simulink model "noxiebo"  (R2018b)
settings: Solver=FixedStepDiscrete  StartTime=0.0  StopTime=Inf  FixedStep=Auto  RelTol=1e-3  EnableMultiTasking=on
model workspace (MAT data in the model file):
  encoderResolution = 4096
  indexOffset = 0
  polePairs = 16
undefined symbols (not defined in the file or in its folder): Down, Up
libraries: idelinklib_common x37, c2833xlib x7, c280xlib x6, simulink x3, simulink_extras x2, c2000lib x1
(part 1 of 3)
settings Model: ExtModeTrigDuration=8  Creator=ChenYu  LastModifiedBy=ThinkPad
settings DataIOCC: LimitDataPoints=on  SaveFormat=Array  SignalLoggingSaveFormat=ModelDataLogs  SaveOutput=off  SaveTime=off
settings OptimizationCC: DefaultUnderspecifiedDataType=single  EnhancedBackFolding=on  PassReuseOutputArgsAs=Individual arguments  ExpressionDepthLimit=2147483647  MaxStackSize=512  OptimizeBlockOrder=speed  DifferentSizesBufferReuse=on  OptimizationCustomize=off
settings DebuggingCC: UnderspecifiedInitializationDetection=Classic  MergeDetectMultiDrivingBlocksExec=none  SolverPrmCheckMsg=warning  ParameterTunabilityLossMsg=error  FcnCallInpInsideContextMsg=warning  StateNameClashWarn=warning  SFUnexpectedBacktrackingDiag=warning  SFNoUnconditionalDefaultTransitionDiag=warning  SFExecutionAtInitializationDiag=none
settings HardwareCC: ProdBitPerChar=16  ProdBitPerInt=16  ProdBitPerPointer=32  ProdBitPerSizeT=32  ProdBitPerPtrDiffT=32  ProdLargestAtomicInteger=Integer  ProdLargestAtomicFloat=None  ProdWordSize=16  ProdLongLongMode=on  ProdHWDeviceType=Texas Instruments->C2000
settings ModelReferenceCC: PropagateSignalLabelsOutOfModel=off
settings SFSimCC: SimUseLocalCustomCode=off  MATLABDynamicMemAlloc=off
settings RTWCC: SystemTargetFile=ert.tlc  HardwareBoard=TI Delfino F2833x  GenCodeOnly=on  TemplateMakefile=ert_default_tmf  GenerateReport=on  RTWUseLocalCustomCode=off  Toolchain=Texas Instruments Code Composer Studio (C2000)  IncludeHyperlinkInReport=on  LaunchReport=on  GenerateTraceInfo=on  GenerateTraceReport=on  GenerateTraceReportSl=on  GenerateTraceReportSf=on  GenerateTraceReportEml=on
settings RTWCC: CustomInitializer=|
  | // Make sure the XINTF clock is enabled   cool
  | 	SysCtrlRegs.PCLKCR3.bit.XINTFENCLK = 1;
  | 
  | 	// Configure the GPIO for XINTF with a 16-bit data bus
  | 	// This function is in DSP2833x_Xintf.c
  | 	//InitXintf16Gpio();
  | 
  |     EALLOW;
  |     // All Zones---------------------------------
  |     // Timing for all zones based on XTIMCLK = SYSCLKOUT/2
  |     XintfRegs.XINTCNF2.bit.XTIMCLK = 1;
  |     // Buffer up to 3 writes
  |     XintfRegs.XINTCNF2.bit.WRBUFF = 3;
  |     // XCLKOUT is enabled
  |     XintfRegs.XINTCNF2.bit.CLKOFF = 0;
  |     // XCLKOUT = XTIMCLK/2
  |     XintfRegs.XINTCNF2.bit.CLKMODE = 1;
  | 
  |     // Zone 7------------------------------------
  |     // When using ready, ACTIVE must be 1 or greater
  |     // Lead must always be 1 or greater
  |     // Zone write timing
  |     XintfRegs.XTIMING7.bit.XWRLEAD = 3;//3*2*2*SYSCLKOUT
  |     XintfRegs.XTIMING7.bit.XWRACTIVE = 7; //(7+1)*2*2*SYSCLKOUT
  |     XintfRegs.XTIMING7.bit.XWRTRAIL = 3;
  |     // Zone read timing
  |     XintfRegs.XTIMING7.bit.XRDLEAD = 3;
  |     XintfRegs.XTIMING7.bit.XRDACTIVE = 7;
  |     XintfRegs.XTIMING7.bit.XRDTRAIL = 3;
  | 
  |     // double all Zone read/write lead/active/trail timing
  |     XintfRegs.XTIMING7.bit.X2TIMING = 1;
  | 
  |     // Zone will not sample XREADY signal
  |     XintfRegs.XTIMING7.bit.USEREADY = 0;
  |     XintfRegs.XTIMING7.bit.READYMODE = 0;
  | 
  |     // Size must be either:
  |     // 0,1 = x32 or
  |     // 1,1 = x16 other values are reserved
  |     XintfRegs.XTIMING7.bit.XSIZE = 3;
  | 
  |     EDIS;
  | 
  |    //Force a pipeline flush to ensure that the write to
  |    //the last register configured occurs before returning.
  |    asm(" RPT #7 || NOP");
settings CodeAppCC: ForceParamTrailComments=on  IgnoreCustomStorageClasses=off  OperatorAnnotations=on  SimulinkDataObjDesc=on  SFDataObjDesc=on  CustomSymbolStrType=$N$R$M  InsertBlockDesc=on  InternalIdentifier=Classic
settings ERTTargetCC: CodeReplacementLibrary=TI C28x
settings ConfigComp: CovMetricSettings=dw  CovHtmlReporting=on  CovSaveCumulativeToWorkspaceVar=on  CovSaveSingleToWorkspaceVar=on  CovExternalEMLEnable=off

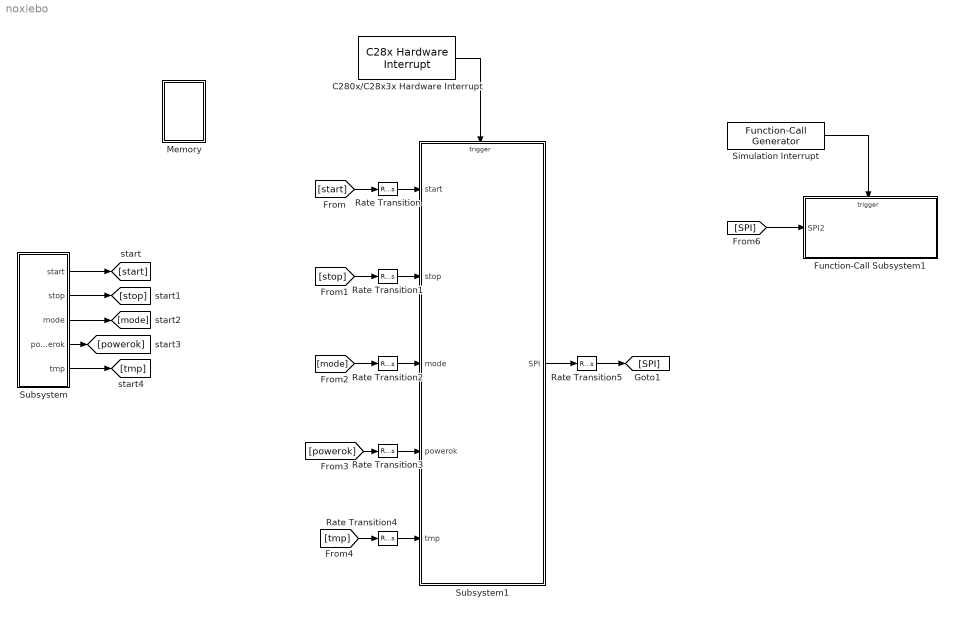
== system noxiebo ==
  C280x/C28x3x Hardware Interrupt : c2000lib/Scheduling/C28x Hardware Interrupt  irqnumbers=[3]  pienumbers=[1]  irqpriorities=[30]  irqpreempts=[0]  showinput=off  dspchiptype=C280X
      settings: SourceProductName=Embedded Coder Support Package for Texas Instruments C2000 Processors  SourceProductBaseCode=TIC2000
  Function-Call Subsystem1 : Subsystem  TreatAsAtomicUnit=on
  Memory : Subsystem
  Rate Transition{,1..5} (6 alike) : RateTransition  Integrity=off
  Simulation Interrupt : simulink/Ports & Subsystems/Function-Call Generator  sample_time=0.005  numberOfIterations=1
  Subsystem : Subsystem
  Subsystem1 : Subsystem
  wires:
  Subsystem/1(start) -> [start]
  Subsystem/2(stop) -> [stop]
  Subsystem/3(mode) -> [mode]
  Subsystem/4(powerok) -> [powerok]
  Subsystem/5(tmp) -> [tmp]
  [start] -> Rate Transition/1
  [stop] -> Rate Transition1/1
  [mode] -> Rate Transition2/1
  [powerok] -> Rate Transition3/1
  [tmp] -> Rate Transition4/1
  Rate Transition/1 -> Subsystem1/1(start)
  Rate Transition1/1 -> Subsystem1/2(stop)
  Rate Transition2/1 -> Subsystem1/3(mode)
  Rate Transition3/1 -> Subsystem1/4(powerok)
  C280x/C28x3x Hardware Interrupt/1 -> Subsystem1/Trigger
  Rate Transition4/1 -> Subsystem1/5(tmp)
  [SPI] -> Function-Call Subsystem1/1(SPI2)
  Simulation Interrupt/1 -> Function-Call Subsystem1/Trigger
  Rate Transition5/1 -> [SPI]
  Subsystem1/1(SPI) -> Rate Transition5/1

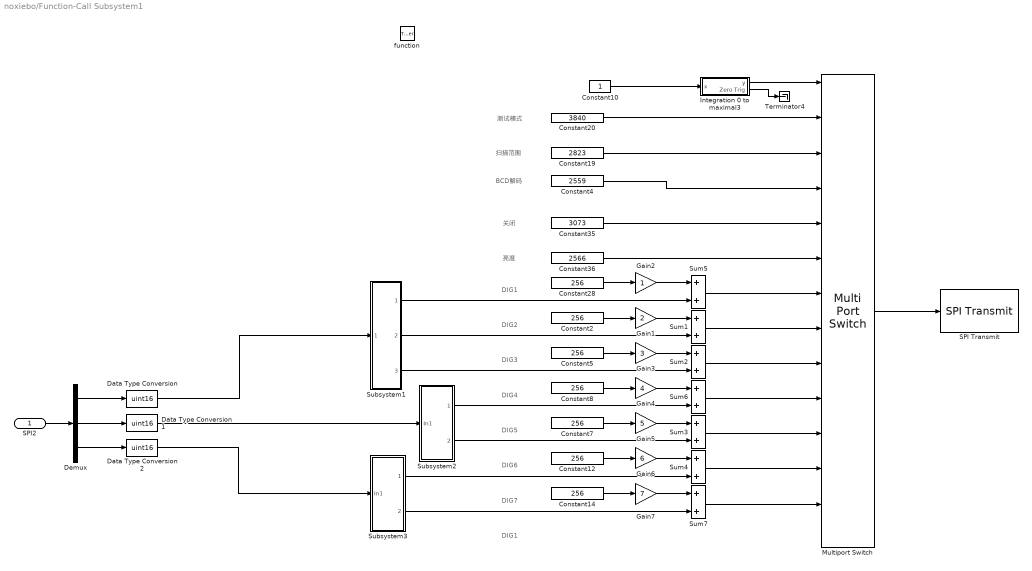
== system noxiebo/Function-Call Subsystem1 ==
  note: 扫描范围
  note: 测试模式
  note: BCD解码
  note: 关闭
  note: 亮度
  note: DIG1
  note: DIG2
  note: DIG3
  note: DIG4
  note: DIG5
  note: DIG6
  note: DIG7
  note: DIG1
  SPI2 : Inport
  function : TriggerPort  TriggerType=function-call  VariantControl=(inherit)
  Constant10 : Constant  OutDataTypeStr=uint16
  Constant{2,5,7..8,12,14,28} (7 alike) : Constant  Value=256  OutDataTypeStr=uint16
  Constant19 : Constant  Value=2823  OutDataTypeStr=uint16
  Constant20 : Constant  Value=3840  OutDataTypeStr=uint16
  Constant35 : Constant  Value=3073  OutDataTypeStr=uint16
  Constant36 : Constant  Value=2566  OutDataTypeStr=uint16
  Constant4 : Constant  Value=2559  OutDataTypeStr=uint16
  Data Type Conversion : DataTypeConversion  OutDataTypeStr=uint16
  Data Type Conversion1 : DataTypeConversion  OutDataTypeStr=uint16
  Data Type Conversion2 : DataTypeConversion  OutDataTypeStr=uint16
  Demux : Demux  Outputs=3
  Gain1 : Gain  Gain=2
  Gain2 : Gain
  Gain3 : Gain  Gain=3
  Gain4 : Gain  Gain=4
  Gain5 : Gain  Gain=5
  Gain6 : Gain  Gain=6
  Gain7 : Gain  Gain=7
  Integration 0 to maximal3 : Subsystem  mask{a=12}
      mask prompts: a "the maximal y"
  Multiport Switch : MultiPortSwitch  Inputs=12  DataPortForDefault=Additional data port  OutDataTypeStr=uint16
  SPI Transmit : c280xlib/SPI Transmit  SPISelect=SPI_A  ClockPolarity=Rising_edge  ClockPhase=No_delay  SPIModule=uint32(0)  Mode=Master  BusSpeed=uint32(1000000)  FirstBitToTransfer=Most significant bit (MSB)  ClockMode=0  BlockFunction=Write  EnableRegisterAddress=on  RegisterAddress=0  OutputDataType=int8  OutputDataLength=1  BlockingMode=off  DataBits=8  UseCustomSSPin=Provided by the SPI peripheral  ActiveLowSSPin=Active low  Pin=0
      settings: SourceProductName=Embedded Coder Support Package for Texas Instruments C2000 Processors  SourceProductBaseCode=TIC2000
  Subsystem1 : Subsystem
  Subsystem2 : Subsystem
  Subsystem3 : Subsystem
  Sum{1..7} (7 alike) : Sum
  Terminator4 : Terminator
  wires:
  Constant10/1 -> Integration 0 to maximal3/1(x)
  Constant19/1 -> Multiport Switch/3
  Constant20/1 -> Multiport Switch/2
  Integration 0 to maximal3/1(y) -> Multiport Switch/1
  Constant35/1 -> Multiport Switch/5
  Constant36/1 -> Multiport Switch/6
  Multiport Switch/1 -> SPI Transmit/1
  Constant28/1 -> Gain2/1
  Sum5/1 -> Multiport Switch/7
  Constant2/1 -> Gain1/1
  Sum1/1 -> Multiport Switch/8
  Constant5/1 -> Gain3/1
  Sum2/1 -> Multiport Switch/9
  Sum6/1 -> Multiport Switch/10
  Subsystem2/1(Out2) -> Sum6/2
  Constant7/1 -> Gain5/1
  Sum3/1 -> Multiport Switch/11
  Subsystem2/2(Out3) -> Sum3/2
  Constant12/1 -> Gain6/1
  Sum4/1 -> Multiport Switch/12
  Subsystem3/1(Out2) -> Sum4/2
  Constant14/1 -> Gain7/1
  Sum7/1 -> Multiport Switch/13
  Gain2/1 -> Sum5/1
  Constant8/1 -> Gain4/1
  Gain1/1 -> Sum1/1
  Gain3/1 -> Sum2/1
  Gain4/1 -> Sum6/1
  Gain5/1 -> Sum3/1
  Gain6/1 -> Sum4/1
  Subsystem3/2(Out3) -> Sum7/2
  Gain7/1 -> Sum7/1
  Constant4/1 -> Multiport Switch/4
  Subsystem1/1(Out1) -> Sum5/2
  Subsystem1/2(Out2) -> Sum1/2
  Subsystem1/3(Out3) -> Sum2/2
  Demux/1 -> Data Type Conversion/1
  Demux/2 -> Data Type Conversion1/1
  Demux/3 -> Data Type Conversion2/1
  SPI2/1 -> Demux/1
  Data Type Conversion/1 -> Subsystem1/1(In1)
  Data Type Conversion1/1 -> Subsystem2/1(In1)
  Data Type Conversion2/1 -> Subsystem3/1(In1)
  Integration 0 to maximal3/2(Zero Trig) -> Terminator4/1

== system noxiebo/Memory ==
  Memory Allocate : idelinklib_common/Memory Allocate  variableName=p1  alignThisVariable=off  memoryAlignmentBoundary=4  dataType=int16  specifyQualifier=off  typeQualifier=volatile  dataDimension=1  specifyMemorySection=off  memorySection=mySEC1  bindMemorySection=off  sectionStartAddress=hex2dec('8000')  initializeMemory=on  initialValue=0
  Memory Allocate1 : idelinklib_common/Memory Allocate  variableName=p2  alignThisVariable=off  memoryAlignmentBoundary=4  dataType=int16  specifyQualifier=off  typeQualifier=volatile  dataDimension=1  specifyMemorySection=off  memorySection=mySEC1  bindMemorySection=off  sectionStartAddress=hex2dec('8000')  initializeMemory=on  initialValue=0
  Memory Allocate10 : idelinklib_common/Memory Allocate  variableName=p11  alignThisVariable=off  memoryAlignmentBoundary=4  dataType=int16  specifyQualifier=off  typeQualifier=volatile  dataDimension=1  specifyMemorySection=off  memorySection=mySEC1  bindMemorySection=off  sectionStartAddress=hex2dec('8000')  initializeMemory=on  initialValue=0
  Memory Allocate11 : idelinklib_common/Memory Allocate  variableName=data1  alignThisVariable=off  memoryAlignmentBoundary=4  dataType=int16  specifyQualifier=off  typeQualifier=volatile  dataDimension=1  specifyMemorySection=off  memorySection=mySEC1  bindMemorySection=off  sectionStartAddress=hex2dec('8000')  initializeMemory=on  initialValue=0
  Memory Allocate12 : idelinklib_common/Memory Allocate  variableName=data2  alignThisVariable=off  memoryAlignmentBoundary=4  dataType=int16  specifyQualifier=off  typeQualifier=volatile  dataDimension=1  specifyMemorySection=off  memorySection=mySEC1  bindMemorySection=off  sectionStartAddress=hex2dec('8000')  initializeMemory=on  initialValue=0
  Memory Allocate13 : idelinklib_common/Memory Allocate  variableName=data3  alignThisVariable=off  memoryAlignmentBoundary=4  dataType=int16  specifyQualifier=off  typeQualifier=volatile  dataDimension=1  specifyMemorySection=off  memorySection=mySEC1  bindMemorySection=off  sectionStartAddress=hex2dec('8000')  initializeMemory=on  initialValue=0
  Memory Allocate14 : idelinklib_common/Memory Allocate  variableName=data4  alignThisVariable=off  memoryAlignmentBoundary=4  dataType=int16  specifyQualifier=off  typeQualifier=volatile  dataDimension=1  specifyMemorySection=off  memorySection=mySEC1  bindMemorySection=off  sectionStartAddress=hex2dec('8000')  initializeMemory=on  initialValue=0
  Memory Allocate15 : idelinklib_common/Memory Allocate  variableName=data5  alignThisVariable=off  memoryAlignmentBoundary=4  dataType=int16  specifyQualifier=off  typeQualifier=volatile  dataDimension=1  specifyMemorySection=off  memorySection=mySEC1  bindMemorySection=off  sectionStartAddress=hex2dec('8000')  initializeMemory=on  initialValue=0
  Memory Allocate16 : idelinklib_common/Memory Allocate  variableName=data6  alignThisVariable=off  memoryAlignmentBoundary=4  dataType=int16  specifyQualifier=off  typeQualifier=volatile  dataDimension=1  specifyMemorySection=off  memorySection=mySEC1  bindMemorySection=off  sectionStartAddress=hex2dec('8000')  initializeMemory=on  initialValue=0
  Memory Allocate17 : idelinklib_common/Memory Allocate  variableName=data7  alignThisVariable=off  memoryAlignmentBoundary=4  dataType=int16  specifyQualifier=off  typeQualifier=volatile  dataDimension=1  specifyMemorySection=off  memorySection=mySEC1  bindMemorySection=off  sectionStartAddress=hex2dec('8000')  initializeMemory=on  initialValue=0
  Memory Allocate18 : idelinklib_common/Memory Allocate  variableName=data8  alignThisVariable=off  memoryAlignmentBoundary=4  dataType=int16  specifyQualifier=off  typeQualifier=volatile  dataDimension=1  specifyMemorySection=off  memorySection=mySEC1  bindMemorySection=off  sectionStartAddress=hex2dec('8000')  initializeMemory=on  initialValue=0
  Memory Allocate19 : idelinklib_common/Memory Allocate  variableName=data9  alignThisVariable=off  memoryAlignmentBoundary=4  dataType=int16  specifyQualifier=off  typeQualifier=volatile  dataDimension=1  specifyMemorySection=off  memorySection=mySEC1  bindMemorySection=off  sectionStartAddress=hex2dec('8000')  initializeMemory=on  initialValue=0
  Memory Allocate2 : idelinklib_common/Memory Allocate  variableName=p3  alignThisVariable=off  memoryAlignmentBoundary=4  dataType=int16  specifyQualifier=off  typeQualifier=volatile  dataDimension=1  specifyMemorySection=off  memorySection=mySEC1  bindMemorySection=off  sectionStartAddress=hex2dec('8000')  initializeMemory=on  initialValue=0
  Memory Allocate20 : idelinklib_common/Memory Allocate  variableName=data10  alignThisVariable=off  memoryAlignmentBoundary=4  dataType=int16  specifyQualifier=off  typeQualifier=volatile  dataDimension=1  specifyMemorySection=off  memorySection=mySEC1  bindMemorySection=off  sectionStartAddress=hex2dec('8000')  initializeMemory=on  initialValue=0
  Memory Allocate21 : idelinklib_common/Memory Allocate  variableName=data11  alignThisVariable=off  memoryAlignmentBoundary=4  dataType=int16  specifyQualifier=off  typeQualifier=volatile  dataDimension=1  specifyMemorySection=off  memorySection=mySEC1  bindMemorySection=off  sectionStartAddress=hex2dec('8000')  initializeMemory=on  initialValue=0
  Memory Allocate22 : idelinklib_common/Memory Allocate  variableName=data12  alignThisVariable=off  memoryAlignmentBoundary=4  dataType=int16  specifyQualifier=off  typeQualifier=volatile  dataDimension=1  specifyMemorySection=off  memorySection=mySEC1  bindMemorySection=off  sectionStartAddress=hex2dec('8000')  initializeMemory=on  initialValue=0
  Memory Allocate3 : idelinklib_common/Memory Allocate  variableName=p4  alignThisVariable=off  memoryAlignmentBoundary=4  dataType=int16  specifyQualifier=off  typeQualifier=volatile  dataDimension=1  specifyMemorySection=off  memorySection=mySEC1  bindMemorySection=off  sectionStartAddress=hex2dec('8000')  initializeMemory=on  initialValue=0
  Memory Allocate4 : idelinklib_common/Memory Allocate  variableName=p5  alignThisVariable=off  memoryAlignmentBoundary=4  dataType=int16  specifyQualifier=off  typeQualifier=volatile  dataDimension=1  specifyMemorySection=off  memorySection=mySEC1  bindMemorySection=off  sectionStartAddress=hex2dec('8000')  initializeMemory=on  initialValue=0
  Memory Allocate5 : idelinklib_common/Memory Allocate  variableName=p6  alignThisVariable=off  memoryAlignmentBoundary=4  dataType=int16  specifyQualifier=off  typeQualifier=volatile  dataDimension=1  specifyMemorySection=off  memorySection=mySEC1  bindMemorySection=off  sectionStartAddress=hex2dec('8000')  initializeMemory=on  initialValue=0
  Memory Allocate6 : idelinklib_common/Memory Allocate  variableName=p7  alignThisVariable=off  memoryAlignmentBoundary=4  dataType=int16  specifyQualifier=off  typeQualifier=volatile  dataDimension=1  specifyMemorySection=off  memorySection=mySEC1  bindMemorySection=off  sectionStartAddress=hex2dec('8000')  initializeMemory=on  initialValue=0
  Memory Allocate7 : idelinklib_common/Memory Allocate  variableName=p8  alignThisVariable=off  memoryAlignmentBoundary=4  dataType=int16  specifyQualifier=off  typeQualifier=volatile  dataDimension=1  specifyMemorySection=off  memorySection=mySEC1  bindMemorySection=off  sectionStartAddress=hex2dec('8000')  initializeMemory=on  initialValue=0
  Memory Allocate8 : idelinklib_common/Memory Allocate  variableName=p9  alignThisVariable=off  memoryAlignmentBoundary=4  dataType=int16  specifyQualifier=off  typeQualifier=volatile  dataDimension=1  specifyMemorySection=off  memorySection=mySEC1  bindMemorySection=off  sectionStartAddress=hex2dec('8000')  initializeMemory=on  initialValue=0
  Memory Allocate9 : idelinklib_common/Memory Allocate  variableName=p10  alignThisVariable=off  memoryAlignmentBoundary=4  dataType=int16  specifyQualifier=off  typeQualifier=volatile  dataDimension=1  specifyMemorySection=off  memorySection=mySEC1  bindMemorySection=off  sectionStartAddress=hex2dec('8000')  initializeMemory=on  initialValue=0

== system noxiebo/Subsystem ==
  MODE : c2833xlib/Digital Input  GPIO_Number=GPIO40~GPIO47  GPIO_Bit0=on  GPIO_Bit1=off  GPIO_Bit2=off  GPIO_Bit3=off  GPIO_Bit4=off  GPIO_Bit5=off  GPIO_Bit6=off  GPIO_Bit7=off  sampleTime=-1  dataType=boolean  GPIO_Bit0_Qualification=Sync to SYSCLKOUT  GPIO_Bit1_Qualification=Sync to SYSCLKOUT  GPIO_Bit2_Qualification=Sync to SYSCLKOUT  GPIO_Bit3_Qualification=Sync to SYSCLKOUT  GPIO_Bit4_Qualification=Sync to SYSCLKOUT  GPIO_Bit5_Qualification=Sync to SYSCLKOUT  GPIO_Bit6_Qualification=Sync to SYSCLKOUT  GPIO_Bit7_Qualification=Sync to SYSCLKOUT  Qualification_Period=-1
      settings: SourceProductName=Embedded Coder Support Package for Texas Instruments C2000 Processors  SourceProductBaseCode=TIC2000
  MODE1 : c2833xlib/Digital Input  GPIO_Number=GPIO32~GPIO39  GPIO_Bit0=off  GPIO_Bit1=on  GPIO_Bit2=off  GPIO_Bit3=off  GPIO_Bit4=off  GPIO_Bit5=off  GPIO_Bit6=off  GPIO_Bit7=off  sampleTime=-1  dataType=boolean  GPIO_Bit0_Qualification=Sync to SYSCLKOUT  GPIO_Bit1_Qualification=Sync to SYSCLKOUT  GPIO_Bit2_Qualification=Sync to SYSCLKOUT  GPIO_Bit3_Qualification=Sync to SYSCLKOUT  GPIO_Bit4_Qualification=Sync to SYSCLKOUT  GPIO_Bit5_Qualification=Sync to SYSCLKOUT  GPIO_Bit6_Qualification=Sync to SYSCLKOUT  GPIO_Bit7_Qualification=Sync to SYSCLKOUT  Qualification_Period=-1
      settings: SourceProductName=Embedded Coder Support Package for Texas Instruments C2000 Processors  SourceProductBaseCode=TIC2000
  MODE2 : c2833xlib/Digital Input  GPIO_Number=GPIO32~GPIO39  GPIO_Bit0=on  GPIO_Bit1=off  GPIO_Bit2=off  GPIO_Bit3=off  GPIO_Bit4=off  GPIO_Bit5=off  GPIO_Bit6=off  GPIO_Bit7=off  sampleTime=-1  dataType=boolean  GPIO_Bit0_Qualification=Sync to SYSCLKOUT  GPIO_Bit1_Qualification=Sync to SYSCLKOUT  GPIO_Bit2_Qualification=Sync to SYSCLKOUT  GPIO_Bit3_Qualification=Sync to SYSCLKOUT  GPIO_Bit4_Qualification=Sync to SYSCLKOUT  GPIO_Bit5_Qualification=Sync to SYSCLKOUT  GPIO_Bit6_Qualification=Sync to SYSCLKOUT  GPIO_Bit7_Qualification=Sync to SYSCLKOUT  Qualification_Period=-1
      settings: SourceProductName=Embedded Coder Support Package for Texas Instruments C2000 Processors  SourceProductBaseCode=TIC2000
  PB-OFF : c2833xlib/Digital Input  GPIO_Number=GPIO32~GPIO39  GPIO_Bit0=off  GPIO_Bit1=off  GPIO_Bit2=on  GPIO_Bit3=off  GPIO_Bit4=off  GPIO_Bit5=off  GPIO_Bit6=off  GPIO_Bit7=off  sampleTime=-1  dataType=boolean  GPIO_Bit0_Qualification=Sync to SYSCLKOUT  GPIO_Bit1_Qualification=Sync to SYSCLKOUT  GPIO_Bit2_Qualification=Sync to SYSCLKOUT  GPIO_Bit3_Qualification=Sync to SYSCLKOUT  GPIO_Bit4_Qualification=Sync to SYSCLKOUT  GPIO_Bit5_Qualification=Sync to SYSCLKOUT  GPIO_Bit6_Qualification=Sync to SYSCLKOUT  GPIO_Bit7_Qualification=Sync to SYSCLKOUT  Qualification_Period=-1
      settings: SourceProductName=Embedded Coder Support Package for Texas Instruments C2000 Processors  SourceProductBaseCode=TIC2000
  PB-ON : c2833xlib/Digital Input  GPIO_Number=GPIO32~GPIO39  GPIO_Bit0=off  GPIO_Bit1=off  GPIO_Bit2=off  GPIO_Bit3=on  GPIO_Bit4=off  GPIO_Bit5=off  GPIO_Bit6=off  GPIO_Bit7=off  sampleTime=-1  dataType=boolean  GPIO_Bit0_Qualification=Sync to SYSCLKOUT  GPIO_Bit1_Qualification=Sync to SYSCLKOUT  GPIO_Bit2_Qualification=Sync to SYSCLKOUT  GPIO_Bit3_Qualification=Sync to SYSCLKOUT  GPIO_Bit4_Qualification=Sync to SYSCLKOUT  GPIO_Bit5_Qualification=Sync to SYSCLKOUT  GPIO_Bit6_Qualification=Sync to SYSCLKOUT  GPIO_Bit7_Qualification=Sync to SYSCLKOUT  Qualification_Period=-1
      settings: SourceProductName=Embedded Coder Support Package for Texas Instruments C2000 Processors  SourceProductBaseCode=TIC2000
  start : Outport
  stop : Outport  Port=2
  mode : Outport  Port=3
  powerok : Outport  Port=4
  tmp : Outport  Port=5
  wires:
  PB-ON/1 -> start/1
  PB-OFF/1 -> stop/1
  MODE/1 -> mode/1
  MODE1/1 -> powerok/1
  MODE2/1 -> tmp/1

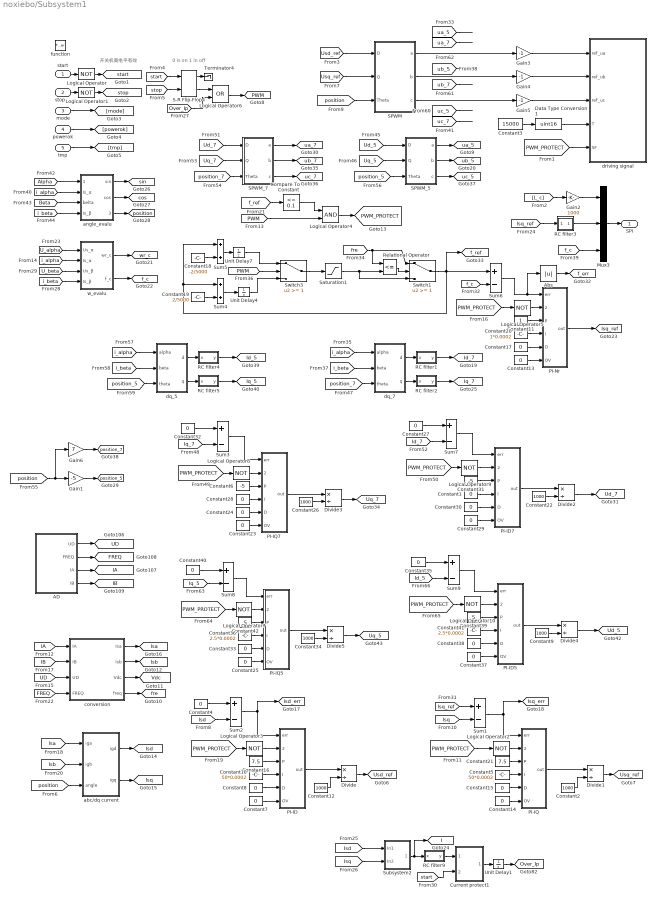
== system noxiebo/Subsystem1 ==
  note: 开关机高电平有效
  note: 0 is on 1 in off
  start : Inport
  stop : Inport  Port=2
  mode : Inport  Port=3
  powerok : Inport  Port=4
  tmp : Inport  Port=5
  function : TriggerPort  TriggerType=function-call  VariantControl=(inherit)
  AD : Subsystem
  Abs : Abs
  Compare To Constant : simulink/Logic and Bit Operations/Compare To Constant  relop=<=  const=0.1  OutDataTypeStr=boolean
  Constant{1,4,7..8,13..15,17,23..25,27..30,32..33,35,37..38,40} (21 alike) : Constant  Value=0  OutDataTypeStr=double
  Constant10 : Constant  Value=50*0.0002  OutDataTypeStr=double
  Constant11 : Constant  OutDataTypeStr=double
  Constant{2,9,12,22,26,34} (6 alike) : Constant  Value=1000  OutDataTypeStr=double
  Constant16 : Constant  Value=7.5  OutDataTypeStr=double
  Constant18 : Constant  Value=-2/5000  OutDataTypeStr=double
  Constant19 : Constant  Value=2/5000  OutDataTypeStr=double
  Constant20 : Constant  Value=1*0.0002  OutDataTypeStr=double
  Constant21 : Constant  Value=7.5  OutDataTypeStr=double
  Constant3 : Constant  Value=15000  OutDataTypeStr=int16
  Constant31 : Constant  Value=-5  OutDataTypeStr=double
  Constant36 : Constant  Value=2.5*0.0002  OutDataTypeStr=double
  Constant39 : Constant  Value=5  OutDataTypeStr=double
  Constant41 : Constant  Value=2.5*0.0002  OutDataTypeStr=double
  Constant42 : Constant  Value=5  OutDataTypeStr=double
  Constant5 : Constant  Value=50*0.0002  OutDataTypeStr=double
  Constant6 : Constant  Value=-5  OutDataTypeStr=double
  Current protect1 : Subsystem
  Data Type Conversion1 : DataTypeConversion  OutDataTypeStr=uint16
  Divide{,1..5} (6 alike) : Product  Inputs=*/
  Gain1 : Gain  Gain=-5
  Gain2 : Gain  Gain=1000
  Gain3 : Gain  Gain=-1
  Gain4 : Gain  Gain=-1
  Gain5 : Gain  Gain=-1
  Gain6 : Gain  Gain=7
  Logical Operator{,1..3,5,7..10} (9 alike) : Logic  Operator=NOT  AllPortsSameDT=off  OutDataTypeStr=boolean
  Logical Operator4 : Logic  AllPortsSameDT=off  OutDataTypeStr=boolean
  Logical Operator6 : Logic  Operator=OR  AllPortsSameDT=off  OutDataTypeStr=boolean
  Mux3 : Mux  Inputs=3
  PI-ID : Subsystem  mask{ermax=3, ermin=-3, max=500, min=-500}
      mask prompts: ermax "Err max limit"; ermin "Err min limit"; max "Output max limit"; min "Output min limit"
  PI-ID5 : Subsystem  mask{ermax=3, ermin=-3, max=500, min=-500}
      mask prompts: ermax "Err max limit"; ermin "Err min limit"; max "Output max limit"; min "Output min limit"
  PI-ID7 : Subsystem  mask{ermax=3, ermin=-3, max=500, min=-500}
      mask prompts: ermax "Err max limit"; ermin "Err min limit"; max "Output max limit"; min "Output min limit"
  PI-IQ : Subsystem  mask{ermax=3, ermin=-3, max=500, min=-500}
      mask prompts: ermax "Err max limit"; ermin "Err min limit"; max "Output max limit"; min "Output min limit"
  PI-IQ5 : Subsystem  mask{ermax=3, ermin=-3, max=500, min=-500}
      mask prompts: ermax "Err max limit"; ermin "Err min limit"; max "Output max limit"; min "Output min limit"
  PI-IQ7 : Subsystem  mask{ermax=3, ermin=-3, max=500, min=-500}
      mask prompts: ermax "Err max limit"; ermin "Err min limit"; max "Output max limit"; min "Output min limit"
  PI-Nr : Subsystem  mask{ermax=15, ermin=-15, max=50, min=0}
      mask prompts: ermax "Err max limit"; ermin "Err min limit"; max "Output max limit"; min "Output min limit"
  RC filter1 : Subsystem  mask{a=0.005}
      mask prompts: a "Time Constant"
  RC filter2 : Subsystem  mask{a=0.005}
      mask prompts: a "Time Constant"
  RC filter3 : Subsystem  mask{a=0.1}
      mask prompts: a "Time Constant"
  RC filter4 : Subsystem  mask{a=0.005}
      mask prompts: a "Time Constant"
  RC filter5 : Subsystem  mask{a=0.005}
      mask prompts: a "Time Constant"
  RC filter9 : Subsystem  mask{a=0.5}
      mask prompts: a "Time Constant"
  Relational Operator : RelationalOperator  Operator=<=  OutDataTypeStr=boolean  RndMeth=Nearest
  S-R Flip-Flop4 : simulink_extras/Flip Flops/S-R Flip-Flop  initial_condition=0
  SPWM : Subsystem
  SPWM_5 : Subsystem
  SPWM_7 : Subsystem
  Saturation1 : Saturate  UpperLimit=40  LowerLimit=0  LinearizeAsGain=off  ZeroCross=off  OutDataTypeStr=double
  Subsystem2 : Subsystem
  Sum{1..3,6..9} (7 alike) : Sum  Inputs=+-
  Sum4 : Sum
  Sum5 : Sum
  Switch1 : Switch  Threshold=1
  Switch3 : Switch  Threshold=1
  Terminator4 : Terminator
  Unit Delay1 : UnitDelay  SampleTime=-1
  Unit Delay4 : UnitDelay  SampleTime=-1
  Unit Delay7 : UnitDelay  SampleTime=-1
  abc/dq current : Subsystem
  angle_evalu : Subsystem
  conversion : Subsystem
  dq_5 : Subsystem
  dq_7 : Subsystem
  driving signal : Subsystem
  w_evalu : Subsystem
  SPI : Outport
  tag scope: FREQ=global, I=global, IA=global, IB=global, Id_5=global, Id_7=global, Iq_5=global, Iq_7=global, Isa=global, Isb=global, Isd=global, Isd_err=global, Isq=global, Isq_err=global, Isq_ref=global, Over_Ip=global, PWM=global, PWM_PROTECT=global, UD=global, Ud_5=global, Ud_7=global, Uq_5=global, Uq_7=global, Usd_ref=global, Usq_ref=global, Vdc=global, cos=global, f_c=global, f_err=global, f_ref=global, fre=global, position=global, position_5=global, position_7=global, sin=global, start=global, stop=global, ua_5=global, ua_7=global, ub_5=global, ub_7=global, uc_5=global, uc_7=global, wr_c=global
  wires:
  Constant3/1 -> Data Type Conversion1/1
  start/1 -> Logical Operator/1
  stop/1 -> Logical Operator1/1
  mode/1 -> [mode]
  powerok/1 -> [powerok]
  tmp/1 -> [tmp]
  Logical Operator/1 -> [start]
  Logical Operator1/1 -> [stop]
  [start] -> S-R Flip-Flop4/1
  [stop] -> S-R Flip-Flop4/2
  S-R Flip-Flop4/1 -> Terminator4/1
  Data Type Conversion1/1 -> driving signal/4(T)
  [PWM_PROTECT] -> driving signal/5(SF)
  [Usd_ref] -> SPWM/1(D)
  [Usq_ref] -> SPWM/2(Q)
  [position] -> SPWM/3(Theta)
  [f_ref] -> Compare To Constant/1
  [PWM] -> Logical Operator4/2
  Compare To Constant/1 -> Logical Operator4/1
  Logical Operator4/1 -> [PWM_PROTECT]
  Gain4/1 -> driving signal/2(ref_ub)
  Gain3/1 -> driving signal/1(ref_ua)
  Gain5/1 -> driving signal/3(ref_uc)
  [PWM_PROTECT] -> Logical Operator3/1
  Constant7/1 -> PI-ID/6(OV)
  Constant8/1 -> PI-ID/5(D)
  Constant10/1 -> PI-ID/4(I)
  Constant16/1 -> PI-ID/3(P)
  Sum2/1 -> [Isd_err], PI-ID/1(err)
  PI-ID/1(out) -> Divide/1
  Divide/1 -> [Usd_ref]
  Constant12/1 -> Divide/2
  Logical Operator2/1 -> PI-IQ/2(reset)
  Constant14/1 -> PI-IQ/6(OV)
  Constant15/1 -> PI-IQ/5(D)
  Constant5/1 -> PI-IQ/4(I)
  Constant21/1 -> PI-IQ/3(P)
  [Isq] -> Sum1/2
  Sum1/1 -> [Isq_err], PI-IQ/1(err)
  [PWM_PROTECT] -> Logical Operator2/1
  Logical Operator3/1 -> PI-ID/2(reset)
  AD/1(UD) -> [UD]
  AD/4(IB) -> [IB]
  AD/3(IA) -> [IA]
  AD/2(FREQ) -> [FREQ]
  conversion/1(Isa) -> [Isa]
  conversion/2(Isb) -> [Isb]
  [IB] -> conversion/2(IB)
  [IA] -> conversion/1(IA)
  [UD] -> conversion/3(UD)
  conversion/3(Vdc) -> [Vdc]
  [Isa] -> abc/dq current/1(iga)
  [Isb] -> abc/dq current/2(igb)
  [position] -> abc/dq current/3(angle)
  abc/dq current/1(igd) -> [Isd]
  abc/dq current/2(igq) -> [Isq]
  PI-IQ/1(out) -> Divide1/1
  Divide1/1 -> [Usq_ref]
  Constant2/1 -> Divide1/2
  [FREQ] -> conversion/4(FREQ)
  conversion/4(freq) -> [fre]
  [Isd] -> Sum2/2
  [Isd] -> Subsystem2/1(In1)
  [Isq] -> Subsystem2/2(In2)
  RC filter9/1(y) -> Current protect1/1(igdin)
  Subsystem2/1(Out1) -> RC filter9/1(x), [I]
  [start] -> Current protect1/2(reset)
  Unit Delay1/1 -> [Over_Ip]
  Current protect1/1(Software_I) -> Unit Delay1/1
  [Over_Ip] -> Logical Operator6/2
  S-R Flip-Flop4/2 -> Logical Operator6/1
  Logical Operator6/1 -> [PWM]
  [i_alpha] -> w_evalu/2(Is_α)
  [U_alpha] -> w_evalu/1(Us_α)
  [i_beta] -> w_evalu/4(Is_β)
  [U_beta] -> w_evalu/3(Us_β)
  w_evalu/1(wr_c) -> [wr_c]
  Mux3/1 -> SPI/1
  [Alpha] -> angle_evalu/1(alpha)
  [Beta] -> angle_evalu/3(belta)
  [i_beta] -> angle_evalu/4(Is_β)
  [i_alpha] -> angle_evalu/2(Is_α)
  angle_evalu/1(sin) -> [sin]
  angle_evalu/2(cos) -> [cos]
  angle_evalu/3(angle_c) -> [position]
  w_evalu/2(f_c) -> [f_c]
  [f_c] -> Mux3/3
  [Isq_ref] -> Sum1/1
  Constant4/1 -> Sum2/1
  [f_c] -> Sum6/2
  Sum6/1 -> PI-Nr/1(err), Abs/1
  [PWM_PROTECT] -> Logical Operator5/1
  Constant13/1 -> PI-Nr/6(OV)
  Constant17/1 -> PI-Nr/5(D)
  Constant20/1 -> PI-Nr/4(I)
  Constant11/1 -> PI-Nr/3(P)
  Logical Operator5/1 -> PI-Nr/2(reset)
  PI-Nr/1(out) -> [Isq_ref]
  Constant18/1 -> Sum5/2
  Sum5/1 -> Unit Delay7/1
  [PWM] -> Switch3/2
  Constant19/1 -> Sum4/2
  Sum4/1 -> Unit Delay4/1
  Unit Delay4/1 -> Switch3/3
  Unit Delay7/1 -> Switch3/1
  [fre] -> Switch1/1, Relational Operator/1
  Switch3/1 -> Saturation1/1
  Relational Operator/1 -> Switch1/2
  Saturation1/1 -> Relational Operator/2, Switch1/3
  Switch1/1 -> Sum5/1, Sum4/1, Sum6/1, [f_ref]
  [L_c] -> Gain2/1
  [Isq_ref] -> RC filter3/1(x)
  Gain2/1 -> Mux3/1
  RC filter3/1(y) -> Mux3/2
  dq_7/1(d) -> RC filter1/1(x)
  [i_alpha] -> dq_7/1(alpha)
  [i_beta] -> dq_7/2(beta)
  [position_7] -> dq_7/3(theta)
  dq_7/2(q) -> RC filter2/1(x)
  [PWM_PROTECT] -> Logical Operator9/1
  Constant29/1 -> PI-ID7/6(OV)
  Constant30/1 -> PI-ID7/5(D)
  Constant1/1 -> PI-ID7/4(I)
  Constant31/1 -> PI-ID7/3(P)
  Sum7/1 -> PI-ID7/1(err)
  PI-ID7/1(out) -> Divide2/1
  Constant22/1 -> Divide2/2
  Logical Operator8/1 -> PI-IQ7/2(reset)
  Constant23/1 -> PI-IQ7/6(OV)
  Constant24/1 -> PI-IQ7/5(D)
  Constant28/1 -> PI-IQ7/4(I)
  Constant6/1 -> PI-IQ7/3(P)
  [Iq_7] -> Sum3/2
  Sum3/1 -> PI-IQ7/1(err)
  [PWM_PROTECT] -> Logical Operator8/1
  Logical Operator9/1 -> PI-ID7/2(reset)
  PI-IQ7/1(out) -> Divide3/1
  Constant26/1 -> Divide3/2
  [Id_7] -> Sum7/2
  Constant32/1 -> Sum3/1
  Constant27/1 -> Sum7/1
  RC filter1/1(y) -> [Id_7]
  RC filter2/1(y) -> [Iq_7]
  [Uq_7] -> SPWM_7/2(Q)
  [Ud_7] -> SPWM_7/1(D)
  [position_7] -> SPWM_7/3(Theta)
  [position] -> Gain1/1, Gain6/1
  Gain1/1 -> [position_5]
  SPWM_7/1(a) -> [ua_7]
  SPWM_7/3(c) -> [uc_7]
  SPWM_7/2(b) -> [ub_7]
  SPWM/1(a) -> Gain3/1
  [ua_5] -> ?
  SPWM/2(b) -> Gain4/1
  [ub_5] -> ?
  SPWM/3(c) -> Gain5/1
  [uc_7] -> ?
  Gain6/1 -> [position_7]
  [ua_7] -> ?
  [uc_5] -> ?
  Abs/1 -> [f_err]
  [ub_7] -> ?
  Divide3/1 -> [Uq_7]
  Divide2/1 -> [Ud_7]
  [Uq_5] -> SPWM_5/2(Q)
  [Ud_5] -> SPWM_5/1(D)
  [position_5] -> SPWM_5/3(Theta)
  SPWM_5/1(a) -> [ua_5]
  SPWM_5/3(c) -> [uc_5]
  SPWM_5/2(b) -> [ub_5]
  dq_5/1(d) -> RC filter4/1(x)
  [i_alpha] -> dq_5/1(alpha)
  [i_beta] -> dq_5/2(beta)
  [position_5] -> dq_5/3(theta)
  dq_5/2(q) -> RC filter5/1(x)
  RC filter4/1(y) -> [Id_5]
  RC filter5/1(y) -> [Iq_5]
  [PWM_PROTECT] -> Logical Operator10/1
  Constant37/1 -> PI-ID5/6(OV)
  Constant38/1 -> PI-ID5/5(D)
  Constant41/1 -> PI-ID5/4(I)
  Constant39/1 -> PI-ID5/3(P)
  Sum9/1 -> PI-ID5/1(err)
  PI-ID5/1(out) -> Divide4/1
  Constant9/1 -> Divide4/2
  Logical Operator7/1 -> PI-IQ5/2(reset)
  Constant25/1 -> PI-IQ5/6(OV)
  Constant33/1 -> PI-IQ5/5(D)
  Constant36/1 -> PI-IQ5/4(I)
  Constant42/1 -> PI-IQ5/3(P)
  [Iq_5] -> Sum8/2
  Sum8/1 -> PI-IQ5/1(err)
  [PWM_PROTECT] -> Logical Operator7/1
  Logical Operator10/1 -> PI-ID5/2(reset)
  PI-IQ5/1(out) -> Divide5/1
  Constant34/1 -> Divide5/2
  [Id_5] -> Sum9/2
  Constant40/1 -> Sum8/1
  Constant35/1 -> Sum9/1
  Divide5/1 -> [Uq_5]
  Divide4/1 -> [Ud_5]

== system noxiebo/Function-Call Subsystem1/Integration 0 to maximal3 ==
  x : Inport
  3 : Constant  Value=a  OutDataTypeStr=fixdt(1,32,16)
  Relational Operator1 : RelationalOperator  Operator=<=  RndMeth=Nearest
  Sum1 : Sum  Inputs=+-
  Sum2 : Sum
  Switch2 : Switch  Criteria=u2 > Threshold  SaturateOnIntegerOverflow=on  InputSameDT=on
  Unit Delay1 : UnitDelay  SampleTime=-1
  y : Outport
  Zero Trig : Outport  Port=2
  wires:
  x/1 -> Sum2/2
  Sum1/1 -> Switch2/3
  Switch2/1 -> y/1, Unit Delay1/1
  Relational Operator1/1 -> Zero Trig/1, Switch2/2
  3/1 -> Sum1/2, Relational Operator1/2
  Sum2/1 -> Sum1/1, Relational Operator1/1, Switch2/1
  Unit Delay1/1 -> Sum2/1

== system noxiebo/Function-Call Subsystem1/Subsystem1 ==
  In1 : Inport
  求个位 : Subsystem
  求十位 : Subsystem
  求百位 : Subsystem
  Out1 : Outport
  Out2 : Outport  Port=2
  Out3 : Outport  Port=3
  wires:
  In1/1 -> 求百位/1(In1), 求十位/2(In2), 求个位/1(In1)
  求个位/1(Out1) -> Out3/1
  求百位/1(Out1) -> Out1/1, 求十位/1(In1), 求个位/2(In2)
  求十位/1(Out1) -> Out2/1, 求个位/3(In3)

== system noxiebo/Function-Call Subsystem1/Subsystem2 ==
  In1 : Inport
  求个位 : Subsystem
  求十位 : Subsystem
  求百位 : Subsystem
  Out2 : Outport
  Out3 : Outport  Port=2
  wires:
  求十位/1(Out1) -> 求个位/3(In3), Out2/1
  求百位/1(Out1) -> 求个位/2(In2), 求十位/1(In1)
  求个位/1(Out1) -> Out3/1
  In1/1 -> 求个位/1(In1), 求十位/2(In2), 求百位/1(In1)

== system noxiebo/Function-Call Subsystem1/Subsystem3 ==
  In1 : Inport
  求个位 : Subsystem
  求十位 : Subsystem
  求百位 : Subsystem
  Out2 : Outport
  Out3 : Outport  Port=2
  wires:
  In1/1 -> 求百位/1(In1), 求十位/2(In2), 求个位/1(In1)
  求个位/1(Out1) -> Out3/1
  求百位/1(Out1) -> 求十位/1(In1), 求个位/2(In2)
  求十位/1(Out1) -> Out2/1, 求个位/3(In3)

== system noxiebo/Subsystem1/AD ==
  Start Conversion : Subsystem  Priority=1
  Stop Conversion : Subsystem  Priority=3
  read AD : Subsystem
  UD : Outport
  FREQ : Outport  Port=2
  IA : Outport  Port=3
  IB : Outport  Port=4
  wires:
  read AD/1(UD) -> UD/1
  read AD/2(UOUT) -> [UOUT]
  read AD/3(UOUT1) -> [UOUT1]
  read AD/4(FREQ) -> FREQ/1
  read AD/5(IA) -> IA/1
  read AD/6(IB) -> IB/1

== system noxiebo/Subsystem1/Current protect1 ==
  igdin : Inport
  reset : Inport  Port=2
  Constant25 : Constant  Value=0  OutDataTypeStr=boolean
  Constant26 : Constant  OutDataTypeStr=boolean
  S-R Flip-Flop1 : simulink_extras/Flip Flops/S-R Flip-Flop  initial_condition=0
  Switch9 : Switch  Criteria=u2 > Threshold  Threshold=120  SaturateOnIntegerOverflow=on  InputSameDT=on
  Terminator : Terminator
  Software_I : Outport
  wires:
  igdin/1 -> Switch9/2
  S-R Flip-Flop1/1 -> Software_I/1
  Constant25/1 -> Switch9/3
  Constant26/1 -> Switch9/1
  S-R Flip-Flop1/2 -> Terminator/1
  Switch9/1 -> S-R Flip-Flop1/1
  reset/1 -> S-R Flip-Flop1/2

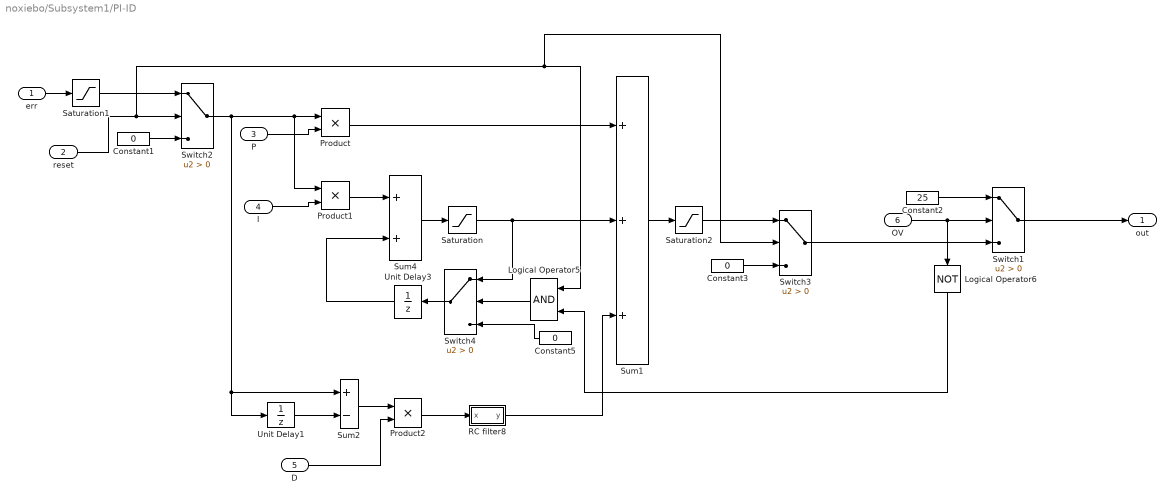
== system noxiebo/Subsystem1/PI-ID ==
  err : Inport
  reset : Inport  Port=2
  P : Inport  Port=3
  I : Inport  Port=4
  D : Inport  Port=5
  OV : Inport  Port=6
  Constant1 : Constant  Value=0  OutDataTypeStr=Inherit: Inherit via back propagation
  Constant2 : Constant  Value=25  OutDataTypeStr=Inherit: Inherit via back propagation
  Constant3 : Constant  Value=0  OutDataTypeStr=Inherit: Inherit via back propagation
  Constant5 : Constant  Value=0  OutDataTypeStr=Inherit: Inherit via back propagation
  Logical Operator5 : Logic  AllPortsSameDT=off  OutDataTypeStr=boolean
  Logical Operator6 : Logic  Operator=NOT  AllPortsSameDT=off  OutDataTypeStr=boolean
  Product : Product  RndMeth=Zero
  Product1 : Product  RndMeth=Zero
  Product2 : Product  RndMeth=Zero
  RC filter8 : Subsystem  mask{a=0.4}
      mask prompts: a "Time Constant"
  Saturation : Saturate  UpperLimit=max  LowerLimit=min  LinearizeAsGain=off  ZeroCross=off  OutDataTypeStr=double
  Saturation1 : Saturate  UpperLimit=ermax  LowerLimit=ermin  LinearizeAsGain=off  ZeroCross=off  OutDataTypeStr=double
  Saturation2 : Saturate  UpperLimit=max  LowerLimit=min  LinearizeAsGain=off  ZeroCross=off  OutDataTypeStr=double
  Sum1 : Sum  Inputs=+++
  Sum2 : Sum  Inputs=+-
  Sum4 : Sum
  Switch{1..4} (4 alike) : Switch  Criteria=u2 > Threshold  SaturateOnIntegerOverflow=on  InputSameDT=on
  Unit Delay1 : UnitDelay  SampleTime=-1
  Unit Delay3 : UnitDelay  SampleTime=-1
  out : Outport
  wires:
  Logical Operator6/1 -> Logical Operator5/2
  Logical Operator5/1 -> Switch4/2
  RC filter8/1(y) -> Sum1/3
  Constant3/1 -> Switch3/3
  Switch3/1 -> Switch1/3
  Saturation2/1 -> Switch3/1
  Switch1/1 -> out/1
  OV/1 -> Logical Operator6/1, Switch1/2
  Constant2/1 -> Switch1/1
  Sum1/1 -> Saturation2/1
  Product2/1 -> RC filter8/1(x)
  Unit Delay1/1 -> Sum2/2
  D/1 -> Product2/2
  Sum2/1 -> Product2/1
  Switch4/1 -> Unit Delay3/1
  Unit Delay3/1 -> Sum4/2
  Saturation/1 -> Switch4/1, Sum1/2
  Sum4/1 -> Saturation/1
  Product1/1 -> Sum4/1
  I/1 -> Product1/2
  Product/1 -> Sum1/1
  Saturation1/1 -> Switch2/1
  err/1 -> Saturation1/1
  Constant1/1 -> Switch2/3
  reset/1 -> Logical Operator5/1, Switch3/2, Switch2/2
  Switch2/1 -> Unit Delay1/1, Sum2/1, Product1/1, Product/1
  P/1 -> Product/2
  Constant5/1 -> Switch4/3

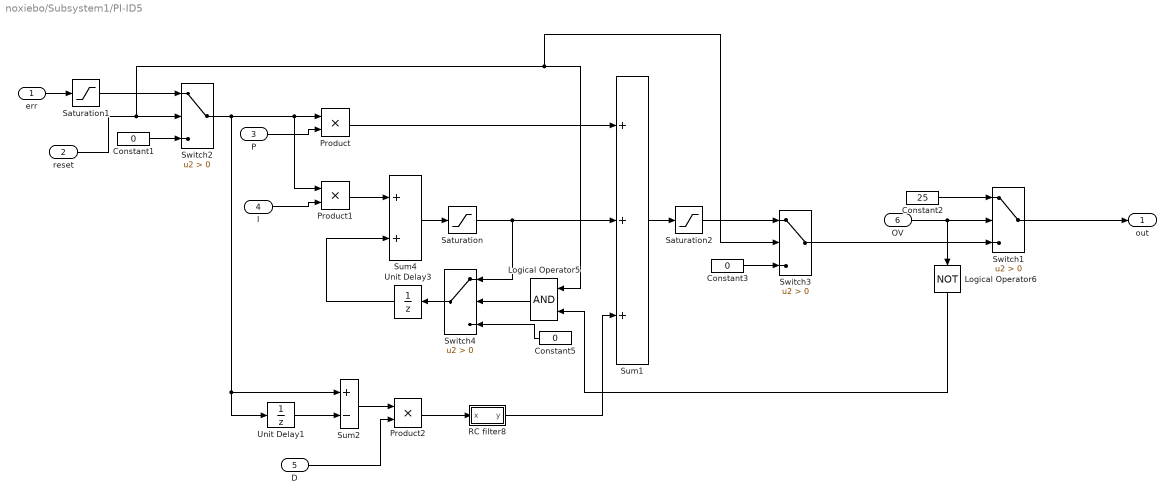
== system noxiebo/Subsystem1/PI-ID5 ==
  err : Inport
  reset : Inport  Port=2
  P : Inport  Port=3
  I : Inport  Port=4
  D : Inport  Port=5
  OV : Inport  Port=6
  Constant1 : Constant  Value=0  OutDataTypeStr=Inherit: Inherit via back propagation
  Constant2 : Constant  Value=25  OutDataTypeStr=Inherit: Inherit via back propagation
  Constant3 : Constant  Value=0  OutDataTypeStr=Inherit: Inherit via back propagation
  Constant5 : Constant  Value=0  OutDataTypeStr=Inherit: Inherit via back propagation
  Logical Operator5 : Logic  AllPortsSameDT=off  OutDataTypeStr=boolean
  Logical Operator6 : Logic  Operator=NOT  AllPortsSameDT=off  OutDataTypeStr=boolean
  Product : Product  RndMeth=Zero
  Product1 : Product  RndMeth=Zero
  Product2 : Product  RndMeth=Zero
  RC filter8 : Subsystem  mask{a=0.4}
      mask prompts: a "Time Constant"
  Saturation : Saturate  UpperLimit=max  LowerLimit=min  LinearizeAsGain=off  ZeroCross=off  OutDataTypeStr=double
  Saturation1 : Saturate  UpperLimit=ermax  LowerLimit=ermin  LinearizeAsGain=off  ZeroCross=off  OutDataTypeStr=double
  Saturation2 : Saturate  UpperLimit=max  LowerLimit=min  LinearizeAsGain=off  ZeroCross=off  OutDataTypeStr=double
  Sum1 : Sum  Inputs=+++
  Sum2 : Sum  Inputs=+-
  Sum4 : Sum
  Switch{1..4} (4 alike) : Switch  Criteria=u2 > Threshold  SaturateOnIntegerOverflow=on  InputSameDT=on
  Unit Delay1 : UnitDelay  SampleTime=-1
  Unit Delay3 : UnitDelay  SampleTime=-1
  out : Outport
  wires:
  Logical Operator6/1 -> Logical Operator5/2
  Logical Operator5/1 -> Switch4/2
  RC filter8/1(y) -> Sum1/3
  Constant3/1 -> Switch3/3
  Switch3/1 -> Switch1/3
  Saturation2/1 -> Switch3/1
  Switch1/1 -> out/1
  OV/1 -> Logical Operator6/1, Switch1/2
  Constant2/1 -> Switch1/1
  Sum1/1 -> Saturation2/1
  Product2/1 -> RC filter8/1(x)
  Unit Delay1/1 -> Sum2/2
  D/1 -> Product2/2
  Sum2/1 -> Product2/1
  Switch4/1 -> Unit Delay3/1
  Unit Delay3/1 -> Sum4/2
  Saturation/1 -> Switch4/1, Sum1/2
  Sum4/1 -> Saturation/1
  Product1/1 -> Sum4/1
  I/1 -> Product1/2
  Product/1 -> Sum1/1
  Saturation1/1 -> Switch2/1
  err/1 -> Saturation1/1
  Constant1/1 -> Switch2/3
  reset/1 -> Logical Operator5/1, Switch3/2, Switch2/2
  Switch2/1 -> Unit Delay1/1, Sum2/1, Product1/1, Product/1
  P/1 -> Product/2
  Constant5/1 -> Switch4/3

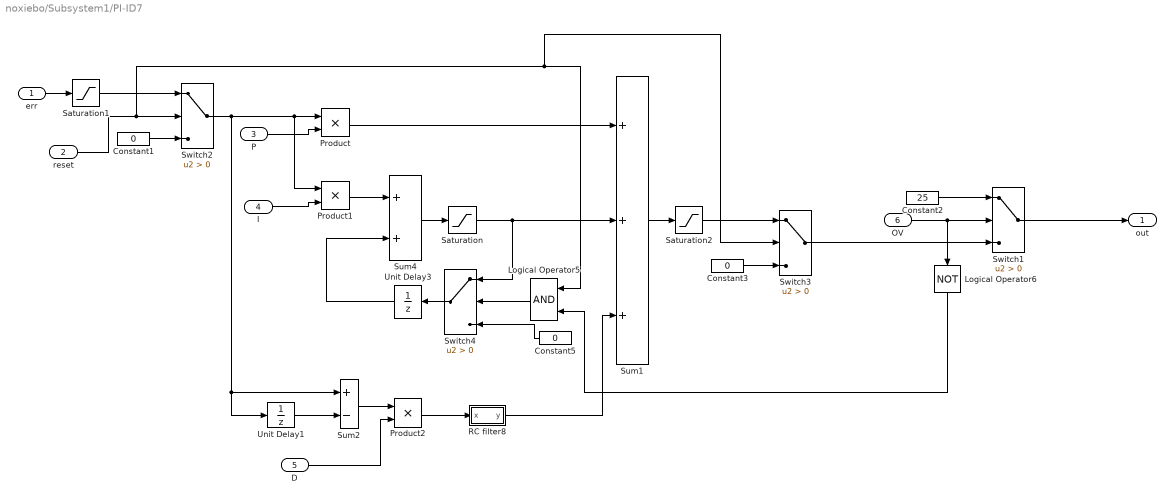
== system noxiebo/Subsystem1/PI-ID7 ==
  err : Inport
  reset : Inport  Port=2
  P : Inport  Port=3
  I : Inport  Port=4
  D : Inport  Port=5
  OV : Inport  Port=6
  Constant1 : Constant  Value=0  OutDataTypeStr=Inherit: Inherit via back propagation
  Constant2 : Constant  Value=25  OutDataTypeStr=Inherit: Inherit via back propagation
  Constant3 : Constant  Value=0  OutDataTypeStr=Inherit: Inherit via back propagation
  Constant5 : Constant  Value=0  OutDataTypeStr=Inherit: Inherit via back propagation
  Logical Operator5 : Logic  AllPortsSameDT=off  OutDataTypeStr=boolean
  Logical Operator6 : Logic  Operator=NOT  AllPortsSameDT=off  OutDataTypeStr=boolean
  Product : Product  RndMeth=Zero
  Product1 : Product  RndMeth=Zero
  Product2 : Product  RndMeth=Zero
  RC filter8 : Subsystem  mask{a=0.4}
      mask prompts: a "Time Constant"
  Saturation : Saturate  UpperLimit=max  LowerLimit=min  LinearizeAsGain=off  ZeroCross=off  OutDataTypeStr=double
  Saturation1 : Saturate  UpperLimit=ermax  LowerLimit=ermin  LinearizeAsGain=off  ZeroCross=off  OutDataTypeStr=double
  Saturation2 : Saturate  UpperLimit=max  LowerLimit=min  LinearizeAsGain=off  ZeroCross=off  OutDataTypeStr=double
  Sum1 : Sum  Inputs=+++
  Sum2 : Sum  Inputs=+-
  Sum4 : Sum
  Switch{1..4} (4 alike) : Switch  Criteria=u2 > Threshold  SaturateOnIntegerOverflow=on  InputSameDT=on
  Unit Delay1 : UnitDelay  SampleTime=-1
  Unit Delay3 : UnitDelay  SampleTime=-1
  out : Outport
  wires:
  Logical Operator6/1 -> Logical Operator5/2
  Logical Operator5/1 -> Switch4/2
  RC filter8/1(y) -> Sum1/3
  Constant3/1 -> Switch3/3
  Switch3/1 -> Switch1/3
  Saturation2/1 -> Switch3/1
  Switch1/1 -> out/1
  OV/1 -> Logical Operator6/1, Switch1/2
  Constant2/1 -> Switch1/1
  Sum1/1 -> Saturation2/1
  Product2/1 -> RC filter8/1(x)
  Unit Delay1/1 -> Sum2/2
  D/1 -> Product2/2
  Sum2/1 -> Product2/1
  Switch4/1 -> Unit Delay3/1
  Unit Delay3/1 -> Sum4/2
  Saturation/1 -> Switch4/1, Sum1/2
  Sum4/1 -> Saturation/1
  Product1/1 -> Sum4/1
  I/1 -> Product1/2
  Product/1 -> Sum1/1
  Saturation1/1 -> Switch2/1
  err/1 -> Saturation1/1
  Constant1/1 -> Switch2/3
  reset/1 -> Logical Operator5/1, Switch3/2, Switch2/2
  Switch2/1 -> Unit Delay1/1, Sum2/1, Product1/1, Product/1
  P/1 -> Product/2
  Constant5/1 -> Switch4/3

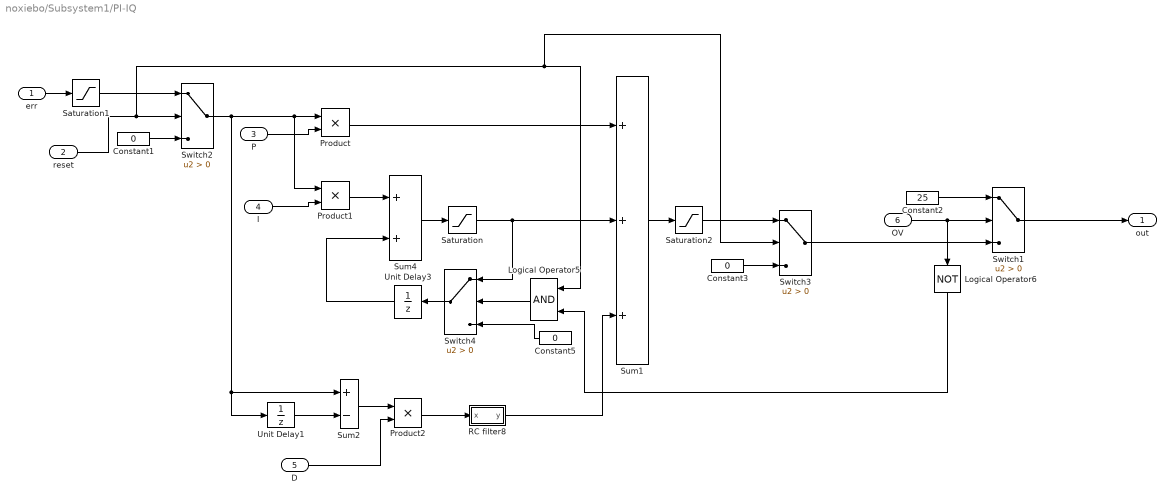
== system noxiebo/Subsystem1/PI-IQ ==
  err : Inport
  reset : Inport  Port=2
  P : Inport  Port=3
  I : Inport  Port=4
  D : Inport  Port=5
  OV : Inport  Port=6
  Constant1 : Constant  Value=0  OutDataTypeStr=Inherit: Inherit via back propagation
  Constant2 : Constant  Value=25  OutDataTypeStr=Inherit: Inherit via back propagation
  Constant3 : Constant  Value=0  OutDataTypeStr=Inherit: Inherit via back propagation
  Constant5 : Constant  Value=0  OutDataTypeStr=Inherit: Inherit via back propagation
  Logical Operator5 : Logic  AllPortsSameDT=off  OutDataTypeStr=boolean
  Logical Operator6 : Logic  Operator=NOT  AllPortsSameDT=off  OutDataTypeStr=boolean
  Product : Product  RndMeth=Zero
  Product1 : Product  RndMeth=Zero
  Product2 : Product  RndMeth=Zero
  RC filter8 : Subsystem  mask{a=0.4}
      mask prompts: a "Time Constant"
  Saturation : Saturate  UpperLimit=max  LowerLimit=min  LinearizeAsGain=off  ZeroCross=off  OutDataTypeStr=double
  Saturation1 : Saturate  UpperLimit=ermax  LowerLimit=ermin  LinearizeAsGain=off  ZeroCross=off  OutDataTypeStr=double
  Saturation2 : Saturate  UpperLimit=max  LowerLimit=min  LinearizeAsGain=off  ZeroCross=off  OutDataTypeStr=double
  Sum1 : Sum  Inputs=+++
  Sum2 : Sum  Inputs=+-
  Sum4 : Sum
  Switch{1..4} (4 alike) : Switch  Criteria=u2 > Threshold  SaturateOnIntegerOverflow=on  InputSameDT=on
  Unit Delay1 : UnitDelay  SampleTime=-1
  Unit Delay3 : UnitDelay  SampleTime=-1
  out : Outport
  wires:
  Constant5/1 -> Switch4/3
  P/1 -> Product/2
  Switch2/1 -> Product/1, Product1/1, Sum2/1, Unit Delay1/1
  reset/1 -> Switch2/2, Switch3/2, Logical Operator5/1
  Constant1/1 -> Switch2/3
  err/1 -> Saturation1/1
  Saturation1/1 -> Switch2/1
  Product/1 -> Sum1/1
  I/1 -> Product1/2
  Product1/1 -> Sum4/1
  Sum4/1 -> Saturation/1
  Saturation/1 -> Sum1/2, Switch4/1
  Unit Delay3/1 -> Sum4/2
  Switch4/1 -> Unit Delay3/1
  Sum2/1 -> Product2/1
  D/1 -> Product2/2
  Unit Delay1/1 -> Sum2/2
  Product2/1 -> RC filter8/1(x)
  Sum1/1 -> Saturation2/1
  Constant2/1 -> Switch1/1
  OV/1 -> Switch1/2, Logical Operator6/1
  Switch1/1 -> out/1
  Saturation2/1 -> Switch3/1
  Switch3/1 -> Switch1/3
  Constant3/1 -> Switch3/3
  RC filter8/1(y) -> Sum1/3
  Logical Operator5/1 -> Switch4/2
  Logical Operator6/1 -> Logical Operator5/2

== system noxiebo/Subsystem1/PI-IQ5 ==
  err : Inport
  reset : Inport  Port=2
  P : Inport  Port=3
  I : Inport  Port=4
  D : Inport  Port=5
  OV : Inport  Port=6
  Constant1 : Constant  Value=0  OutDataTypeStr=Inherit: Inherit via back propagation
  Constant2 : Constant  Value=25  OutDataTypeStr=Inherit: Inherit via back propagation
  Constant3 : Constant  Value=0  OutDataTypeStr=Inherit: Inherit via back propagation
  Constant5 : Constant  Value=0  OutDataTypeStr=Inherit: Inherit via back propagation
  Logical Operator5 : Logic  AllPortsSameDT=off  OutDataTypeStr=boolean
  Logical Operator6 : Logic  Operator=NOT  AllPortsSameDT=off  OutDataTypeStr=boolean
  Product : Product  RndMeth=Zero
  Product1 : Product  RndMeth=Zero
  Product2 : Product  RndMeth=Zero
  RC filter8 : Subsystem  mask{a=0.4}
      mask prompts: a "Time Constant"
  Saturation : Saturate  UpperLimit=max  LowerLimit=min  LinearizeAsGain=off  ZeroCross=off  OutDataTypeStr=double
  Saturation1 : Saturate  UpperLimit=ermax  LowerLimit=ermin  LinearizeAsGain=off  ZeroCross=off  OutDataTypeStr=double
  Saturation2 : Saturate  UpperLimit=max  LowerLimit=min  LinearizeAsGain=off  ZeroCross=off  OutDataTypeStr=double
  Sum1 : Sum  Inputs=+++
  Sum2 : Sum  Inputs=+-
  Sum4 : Sum
  Switch{1..4} (4 alike) : Switch  Criteria=u2 > Threshold  SaturateOnIntegerOverflow=on  InputSameDT=on
  Unit Delay1 : UnitDelay  SampleTime=-1
  Unit Delay3 : UnitDelay  SampleTime=-1
  out : Outport
  wires:
  Constant5/1 -> Switch4/3
  P/1 -> Product/2
  Switch2/1 -> Product/1, Product1/1, Sum2/1, Unit Delay1/1
  reset/1 -> Switch2/2, Switch3/2, Logical Operator5/1
  Constant1/1 -> Switch2/3
  err/1 -> Saturation1/1
  Saturation1/1 -> Switch2/1
  Product/1 -> Sum1/1
  I/1 -> Product1/2
  Product1/1 -> Sum4/1
  Sum4/1 -> Saturation/1
  Saturation/1 -> Sum1/2, Switch4/1
  Unit Delay3/1 -> Sum4/2
  Switch4/1 -> Unit Delay3/1
  Sum2/1 -> Product2/1
  D/1 -> Product2/2
  Unit Delay1/1 -> Sum2/2
  Product2/1 -> RC filter8/1(x)
  Sum1/1 -> Saturation2/1
  Constant2/1 -> Switch1/1
  OV/1 -> Switch1/2, Logical Operator6/1
  Switch1/1 -> out/1
  Saturation2/1 -> Switch3/1
  Switch3/1 -> Switch1/3
  Constant3/1 -> Switch3/3
  RC filter8/1(y) -> Sum1/3
  Logical Operator5/1 -> Switch4/2
  Logical Operator6/1 -> Logical Operator5/2

== system noxiebo/Subsystem1/PI-IQ7 ==
  err : Inport
  reset : Inport  Port=2
  P : Inport  Port=3
  I : Inport  Port=4
  D : Inport  Port=5
  OV : Inport  Port=6
  Constant1 : Constant  Value=0  OutDataTypeStr=Inherit: Inherit via back propagation
  Constant2 : Constant  Value=25  OutDataTypeStr=Inherit: Inherit via back propagation
  Constant3 : Constant  Value=0  OutDataTypeStr=Inherit: Inherit via back propagation
  Constant5 : Constant  Value=0  OutDataTypeStr=Inherit: Inherit via back propagation
  Logical Operator5 : Logic  AllPortsSameDT=off  OutDataTypeStr=boolean
  Logical Operator6 : Logic  Operator=NOT  AllPortsSameDT=off  OutDataTypeStr=boolean
  Product : Product  RndMeth=Zero
  Product1 : Product  RndMeth=Zero
  Product2 : Product  RndMeth=Zero
  RC filter8 : Subsystem  mask{a=0.4}
      mask prompts: a "Time Constant"
  Saturation : Saturate  UpperLimit=max  LowerLimit=min  LinearizeAsGain=off  ZeroCross=off  OutDataTypeStr=double
  Saturation1 : Saturate  UpperLimit=ermax  LowerLimit=ermin  LinearizeAsGain=off  ZeroCross=off  OutDataTypeStr=double
  Saturation2 : Saturate  UpperLimit=max  LowerLimit=min  LinearizeAsGain=off  ZeroCross=off  OutDataTypeStr=double
  Sum1 : Sum  Inputs=+++
  Sum2 : Sum  Inputs=+-
  Sum4 : Sum
  Switch{1..4} (4 alike) : Switch  Criteria=u2 > Threshold  SaturateOnIntegerOverflow=on  InputSameDT=on
  Unit Delay1 : UnitDelay  SampleTime=-1
  Unit Delay3 : UnitDelay  SampleTime=-1
  out : Outport
  wires:
  Constant5/1 -> Switch4/3
  P/1 -> Product/2
  Switch2/1 -> Product/1, Product1/1, Sum2/1, Unit Delay1/1
  reset/1 -> Switch2/2, Switch3/2, Logical Operator5/1
  Constant1/1 -> Switch2/3
  err/1 -> Saturation1/1
  Saturation1/1 -> Switch2/1
  Product/1 -> Sum1/1
  I/1 -> Product1/2
  Product1/1 -> Sum4/1
  Sum4/1 -> Saturation/1
  Saturation/1 -> Sum1/2, Switch4/1
  Unit Delay3/1 -> Sum4/2
  Switch4/1 -> Unit Delay3/1
  Sum2/1 -> Product2/1
  D/1 -> Product2/2
  Unit Delay1/1 -> Sum2/2
  Product2/1 -> RC filter8/1(x)
  Sum1/1 -> Saturation2/1
  Constant2/1 -> Switch1/1
  OV/1 -> Switch1/2, Logical Operator6/1
  Switch1/1 -> out/1
  Saturation2/1 -> Switch3/1
  Switch3/1 -> Switch1/3
  Constant3/1 -> Switch3/3
  RC filter8/1(y) -> Sum1/3
  Logical Operator5/1 -> Switch4/2
  Logical Operator6/1 -> Logical Operator5/2
